simulink model "Model"  (R2021b)
settings: Solver=VariableStepAuto  StartTime=0.0  StopTime=5  RelTol=1e-3
values from neighbouring files (symbols this model uses):
  A = [0 1;9 -1]    [Calculation.m]
  B = [1;0]    [Calculation.m]
  Fb = [-1/(2*r) * (2*p1*b1 + p12*b2), -1/(2*r) * (2*p2*b2 + p12*b1)]    [Calculation.m]
undefined symbols (not defined in the file or in its folder): K
settings Model: Creator=16970  LastModifiedBy=16970

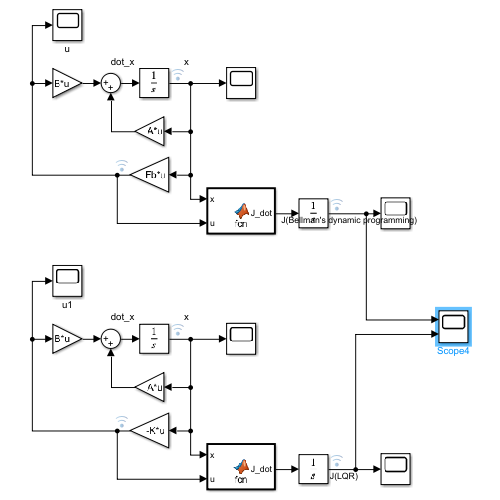
[thumbnail: Simulink's stored preview of the top-level diagram]
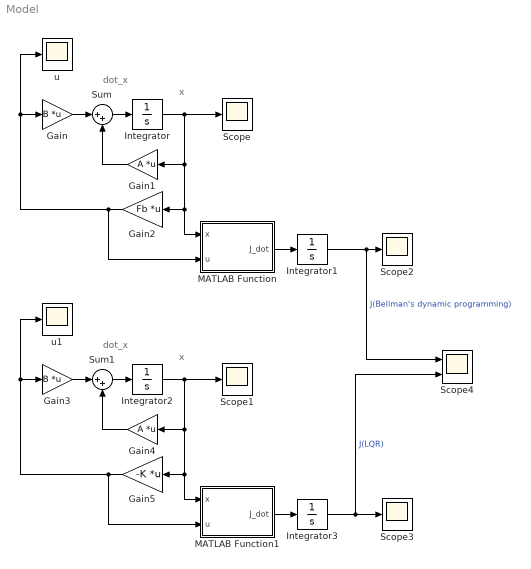
== system Model ==
  note: x
  note: dot_x
  note: x
  note: dot_x
  Gain : Gain  Gain=B  Multiplication=Matrix(K*u)
  Gain1 : Gain  Gain=A  Multiplication=Matrix(K*u)
  Gain2 : Gain  Gain=Fb  Multiplication=Matrix(K*u)
  Gain3 : Gain  Gain=B  Multiplication=Matrix(K*u)
  Gain4 : Gain  Gain=A  Multiplication=Matrix(K*u)
  Gain5 : Gain  Gain=-K  Multiplication=Matrix(K*u)
  Integrator : Integrator  InitialCondition=[1;0]
  Integrator1 : Integrator
  Integrator2 : Integrator  InitialCondition=[1;0]
  Integrator3 : Integrator
  MATLAB Function : MATLAB Function  TreatAsAtomicUnit=on
  MATLAB Function1 : MATLAB Function  TreatAsAtomicUnit=on
  Scope{,1..3} (4 alike) : Scope
  Scope4 : Scope  NumInputPorts=2
  Sum : Sum  Inputs=|++
  Sum1 : Sum  Inputs=|++
  u : Scope
  u1 : Scope
  wires:
  Gain/1 -> Sum/1
  Sum/1 -> Integrator/1
  Integrator/1 -> MATLAB Function/1(x), Gain2/1, Gain1/1, Scope/1
  Gain1/1 -> Sum/2
  Gain2/1 -> MATLAB Function/2(u), u/1, Gain/1
  MATLAB Function/1(J_dot) -> Integrator1/1
  Integrator1/1 -> Scope4/1, Scope2/1  "J(Bellman's dynamic programming)"
  Integrator3/1 -> Scope4/2, Scope3/1  "J(LQR)"
  MATLAB Function1/1(J_dot) -> Integrator3/1
  Gain3/1 -> Sum1/1
  Gain4/1 -> Sum1/2
  Gain5/1 -> MATLAB Function1/2(u), u1/1, Gain3/1
  Integrator2/1 -> MATLAB Function1/1(x), Gain5/1, Gain4/1, Scope1/1
  Sum1/1 -> Integrator2/1

== matlab function Model/MATLAB Function ==
  data: x input; u input; J_dot output
function J_dot = fcn(x, u)
Q = [1 0; 0 2];
r = 1;
%J_acc = 0;
J_dot = x'*Q*x + r*u^2;
%J_acc = J_dot;

end

== matlab function Model/MATLAB Function1 ==
  data: x input; u input; J_dot output
function J_dot = fcn(x, u)
Q = [1 0; 0 2];
r = 1;
%J_acc = 0;
J_dot = x'*Q*x + r*u^2;
%J_acc = J_dot;

end
